simulink model "Ghost_f234"  (Simulink 8.1)
settings: Solver=ode1  StartTime=0.0  StopTime=inf  FixedStep=Ts  MaxStep=1e-3  RelTol=1e-3
PostLoadFcn:
  | NREL_Mode=1; BANSHEE_init;
InitFcn:
  | NREL_Mode=1; BANSHEE_init;
undefined symbols (not defined in the file): CBID, communications_lib, DER_REL, F0, F2, F3, F4, Feeder2_lib, Feeder3_lib, Feeder4_lib, generic_ethernet_cb, Left, relay_housing_lib, SM_UtilityService, SS_COMMUNICATION, SS_F2_RELAY_HOUSING, SS_F3_RELAY_HOUSING, SS_Feeder2, SS_Feeder3, SS_Feeder4, Stim, Ts, type, utility_service_lib, V
libraries: simulink x80, relay_modbus_lib x80, breaker_lib x46, rtio_generic_modbus x45, cables_lib x30, rtlab x22, Load_lib x21, powerlib x20, transformer_lib x19, ssn_lib x13, artemis x6, BESS_lib x4
(part 5 of 6)

== system Ghost_f234/SS_Feeder3/NGCHP_Generator ==
  note: This shall be modbus inputs
  ModbusIn : Inport
  ModbusIn1 : Inport  Port=2
  console : Inport  Port=3
  Heat Load MBtu/hrs : Inport  Port=4
  testseq : Inport  Port=5
  Bus Creator : BusCreator
  Bus Creator2 : BusCreator  Inputs=6
  Bus Creator4 : BusCreator  Inputs=3
  Bus Selector1 : BusSelector  OutputSignals=relay_out  OutputAsBus=on
  Bus Selector2 : BusSelector  OutputSignals=ModbusEnable
  Bus Selector21 : BusSelector  OutputSignals=ModbusFromSC.Ctrl,ModbusFromSC.PCmd,ModbusFromSC.QCmd,ModbusFromSC.VoltCmd,ModbusFromSC.FreqCmd,ModbusFromSC.signal6,ModbusFromSC.signal7,ModbusFromSC.signal8  OutputAsBus=on
  Bus Selector3 : BusSelector  OutputSignals=CHP_SIM_Cmds
  Bus Selector4 : BusSelector  OutputSignals=fault
  Bus Selector5 : BusSelector  OutputSignals=gen2
  Bus Selector6 : BusSelector  OutputSignals=Heat_Recovered_MBtu_hr
  Bus Selector7 : BusSelector  OutputSignals=TempActual,HeatFromBoiler MBtu/hr,CHPHeatContribution MBtu/hr,Thermal data.Heat_Recovered_MBtu_hr,Thermal data.CO2_lbm_hr,Boiler_Nm^3/hr ,Boiler lbm/hr CO2
  Bus to Vector : BusToVector
  CHPThermalModel : CHP_Model_lib/CHPThermalModel  SIM_HIL=SIM_HIL
  Demux : Demux  Outputs=2
  GCB : breaker_lib/Breaker  Ts=Ts  mech_delay=cb_mech_delay
  GenSet : NREL_Diesel_Genset_lib/GenSet  GenSel=3.5MVA natural gas generator
  Generic_Relay : relay_modbus_lib/Generic_Relay_v2_1  Ts=Ts  relay_settings=[DER_REL(CBID.GEN2,:)]
  Mux1 : Mux  Inputs=7
  SimGenCtrl : NREL_Diesel_Genset_lib/Simulated Generator Controller  GenSel=3.5MVA natural gas generator
  Switch : Switch  Criteria=u2 > Threshold  Threshold=0.5
  Gen2 A : PMIOPort  Port=1  Side=Right
  Gen2 B : PMIOPort  Port=2  Side=Right
  Gen2 C : PMIOPort  Port=3  Side=Right
  ModbusOut : Outport
  ModbusOutCHP : Outport  Port=2
  Gen_meas : Outport  Port=3
  wires:
  SimGenCtrl/9 -> Generic_Relay/2  "Logic_trip"
  SimGenCtrl/1 -> ModbusOut/1
  SimGenCtrl/8 -> GenSet/6
  SimGenCtrl/7 -> GenSet/5
  SimGenCtrl/3 -> GenSet/1
  SimGenCtrl/4 -> GenSet/2
  SimGenCtrl/5 -> GenSet/3
  SimGenCtrl/6 -> GenSet/4
  GenSet/1 -> Bus Creator/3  "gen"
  Bus Creator4/1 -> Bus Creator/4, Bus Selector1/1, SimGenCtrl/2  "cb"
  console/1 -> Bus Selector21/1, Bus Selector2/1, Bus Selector3/1
  Bus Selector2/1 -> Switch/2  "<ModbusEnable>"
  ModbusIn/1 -> Switch/1
  Bus Selector21/1 -> Bus to Vector/1
  Bus to Vector/1 -> Switch/3
  Switch/1 -> SimGenCtrl/1
  GCB/1 -> Generic_Relay/1, Bus Creator4/3  "cb_meas"
  Generic_Relay/1 -> Bus Creator4/1  "relay_out"
  Generic_Relay/2 -> Bus Creator4/2  "relay_meas"
  Bus Creator/1 -> Gen_meas/1
  SimGenCtrl/2 -> Bus Creator/2  "ctrl"
  GenSet/2 -> [HeatRec_MBtuhr]
  Bus Selector7/6 -> Mux1/6  "<Boiler_Nm^3/hr >"
  Bus Selector7/7 -> Mux1/7  "<Boiler lbm/hr CO2 >"
  CHPThermalModel/5 -> Bus Creator2/6
  CHPThermalModel/4 -> Bus Creator2/5
  Bus Selector7/3 -> Mux1/3  "<CHPHeatContribution MBtu/hr>"
  CHPThermalModel/1 -> Bus Creator2/2  "TempActual"
  Demux/2 -> CHPThermalModel/4
  CHPThermalModel/2 -> Bus Creator2/3
  Bus Selector7/2 -> Mux1/2  "<HeatFromBoiler MBtu/hr>"
  Bus Selector7/5 -> Mux1/5  "<CO2_lbm_hr>"
  Bus Selector7/4 -> Mux1/4  "<Heat_Recovered_MBtu_hr>"
  Bus Selector7/1 -> Mux1/1  "<TempActual>"
  Heat Load MBtu/hrs/1 -> CHPThermalModel/2
  Mux1/1 -> ModbusOutCHP/1
  Demux/1 -> CHPThermalModel/3
  CHPThermalModel/3 -> Bus Creator2/4
  [HeatRec_MBtuhr] -> Bus Creator2/1, Bus Selector6/1  "Thermal data"
  ModbusIn1/1 -> Demux/1
  Bus Selector6/1 -> CHPThermalModel/1  "<Heat_Recovered_MBtu_hr>"
  Bus Creator2/1 -> Bus Creator/1, Bus Selector7/1  "CHPData"
  Bus Selector3/1 -> CHPThermalModel/5  "<CHP_SIM_Cmds>"
  testseq/1 -> Bus Selector4/1
  Bus Selector4/1 -> Bus Selector5/1  "<fault>"
  Bus Selector5/1 -> SimGenCtrl/3  "<gen2>"
  Bus Selector1/1 -> GCB/1  "<relay_out>"
  connections:
  Gen2 A/RConn1 -- GCB/RConn1
  GCB/RConn2 -- Gen2 B/RConn1
  Gen2 C/RConn1 -- GCB/RConn3
  GenSet/RConn1 -- GCB/LConn1
  GenSet/RConn2 -- GCB/LConn2
  GenSet/RConn3 -- GCB/LConn3

== system Ghost_f234/SS_Feeder4/Diesel_Generator ==
  note: This shall be modbus inputs
  ModbusIn : Inport
  console : Inport  Port=2
  testseq : Inport  Port=3
  phil_meas : Inport  Port=4
  Bus Creator : BusCreator  Inputs=3
  Bus Creator4 : BusCreator  Inputs=3
  Bus Selector1 : BusSelector  OutputSignals=relay_out
  Bus Selector2 : BusSelector  OutputSignals=ModbusEnable
  Bus Selector21 : BusSelector  OutputSignals=ModbusFromSC.Ctrl,ModbusFromSC.PCmd,ModbusFromSC.QCmd,ModbusFromSC.VoltCmd,ModbusFromSC.FreqCmd,ModbusFromSC.signal6,ModbusFromSC.signal7,ModbusFromSC.signal8  OutputAsBus=on
  Bus Selector3 : BusSelector  OutputSignals=fault
  Bus Selector4 : BusSelector  OutputSignals=gen3
  Bus Selector5 : BusSelector  OutputSignals=GEN3_meas,PHIL_Enabled
  Bus to Vector : BusToVector
  GCB : breaker_lib/Breaker  Ts=Ts  mech_delay=cb_mech_delay
  GenSet : NREL_Diesel_Genset_lib/GenSet  GenSel=80kVA diesel generator
  Generic_Relay : relay_modbus_lib/Generic_Relay_v2_1  Ts=Ts  relay_settings=[DER_REL(CBID.GEN3,:)]
  SimGenCtrl : NREL_Diesel_Genset_lib/Simulated Generator Controller  GenSel=80kVA diesel generator
  Switch : Switch  Criteria=u2 > Threshold  Threshold=0.5
  Switch1 : Switch  Threshold=0.5
  Terminator : Terminator
  Gen2 A : PMIOPort  Port=1  Side=Right
  Gen2 B : PMIOPort  Port=2  Side=Right
  Gen2 C : PMIOPort  Port=3  Side=Right
  ModbusOut : Outport
  Gen3 meas : Outport  Port=2
  wires:
  GenSet/2 -> Terminator/1
  SimGenCtrl/2 -> Bus Creator/1  "ctrl"
  Bus Creator/1 -> Gen3 meas/1
  Generic_Relay/2 -> Bus Creator4/2  "relay_meas"
  Generic_Relay/1 -> Bus Creator4/1  "relay_out"
  Switch/1 -> SimGenCtrl/1
  Bus to Vector/1 -> Switch/3
  Bus Selector21/1 -> Bus to Vector/1
  ModbusIn/1 -> Switch/1
  Bus Selector2/1 -> Switch/2  "<ModbusEnable>"
  console/1 -> Bus Selector2/1, Bus Selector21/1
  Bus Creator4/1 -> SimGenCtrl/2, Bus Selector1/1, Bus Creator/3  "cb"
  GenSet/1 -> Bus Creator/2  "gen"
  SimGenCtrl/6 -> GenSet/4
  SimGenCtrl/5 -> GenSet/3
  SimGenCtrl/4 -> GenSet/2
  SimGenCtrl/3 -> GenSet/1
  SimGenCtrl/7 -> GenSet/5
  SimGenCtrl/8 -> GenSet/6
  SimGenCtrl/1 -> ModbusOut/1
  SimGenCtrl/9 -> Generic_Relay/2
  testseq/1 -> Bus Selector3/1
  Bus Selector3/1 -> Bus Selector4/1  "<fault>"
  Bus Selector4/1 -> SimGenCtrl/3  "<gen3>"
  phil_meas/1 -> Bus Selector5/1
  [CB_meas] -> Switch1/3
  Bus Selector5/1 -> Switch1/1  "<GEN3_meas>"
  Bus Selector5/2 -> Switch1/2  "<PHIL_Enabled>"
  GCB/1 -> [CB_meas]  "cb_meas"
  Switch1/1 -> Bus Creator4/3, Generic_Relay/1  "cb_meas"
  Bus Selector1/1 -> GCB/1  "<relay_out>"
  connections:
  GenSet/RConn3 -- GCB/LConn3
  GenSet/RConn2 -- GCB/LConn2
  GenSet/RConn1 -- GCB/LConn1
  Gen2 C/RConn1 -- GCB/RConn3
  GCB/RConn2 -- Gen2 B/RConn1
  Gen2 A/RConn1 -- GCB/RConn1

== system Ghost_f234/SS_Feeder4/ESS2 ==
  modbus_in : Inport
  console : Inport  Port=2
  testseq : Inport  Port=3
  phil_meas : Inport  Port=4
  Bus Creator4 : BusCreator  Inputs=3
  Bus Selector : BusSelector  OutputSignals=cb_ctrl
  Bus Selector1 : BusSelector  OutputSignals=ModbusEnable
  Bus Selector2 : BusSelector  OutputSignals=fault
  Bus Selector20 : BusSelector  OutputSignals=relay_ctrl
  Bus Selector21 : BusSelector  OutputSignals=ModbusFromSC.Ctrl,ModbusFromSC.PCmd,ModbusFromSC.QCmd,ModbusFromSC.VoltCmd,ModbusFromSC.FreqCmd,ModbusFromSC.signal6,ModbusFromSC.signal7,ModbusFromSC.signal8  OutputAsBus=on
  Bus Selector3 : BusSelector  OutputSignals=ess2
  Bus Selector4 : BusSelector  OutputSignals=Tuning
  Bus Selector5 : BusSelector  OutputSignals=ESS2_meas,PHIL_Enabled
  Bus to Vector : BusToVector
  Constant : Constant  Value=0
  ESS2 : BESS_lib/NREL_BESS  InvType=ESS Inverter  Sn=250  Vn=480  b_Vdc_nom=1000  b_kWh=60  b_esr=0.1  r_I_max=3  Tc=Ts  MbusPrecInc=on  ExtTuningEna=on
  F4_CB_3 : breaker_lib/Breaker  Ts=Ts  mech_delay=cb_mech_delay
  Generic_Relay : relay_modbus_lib/Generic_Relay_v2_1  Ts=Ts  relay_settings=[DER_REL(CBID.ESS2,:)]
  Switch : Switch  Criteria=u2 > Threshold  Threshold=0.5
  Switch1 : Switch  Threshold=0.5
  A : PMIOPort  Port=1  Side=Right
  B : PMIOPort  Port=2  Side=Right
  C : PMIOPort  Port=3  Side=Right
  modbus_out : Outport
  meas : Outport  Port=2
  wires:
  Bus Creator4/1 -> ESS2/5
  Generic_Relay/2 -> Bus Creator4/2  "relay_meas"
  ESS2/2 -> meas/1  "PV_meas"
  Generic_Relay/1 -> Bus Creator4/1  "relay_out"
  Bus Selector20/1 -> Generic_Relay/2  "<relay_ctrl>"
  console/1 -> Bus Selector4/1, Bus Selector1/1, Bus Selector21/1
  Bus Selector1/1 -> Switch/2  "<ModbusEnable>"
  ESS2/1 -> modbus_out/1
  modbus_in/1 -> Switch/1
  Bus Selector21/1 -> Bus to Vector/1
  Switch/1 -> ESS2/1
  ESS2/3 -> Bus Selector20/1, Bus Selector/1
  Bus to Vector/1 -> Switch/3
  Constant/1 -> ESS2/3
  testseq/1 -> Bus Selector2/1
  Bus Selector2/1 -> Bus Selector3/1  "<fault>"
  Bus Selector3/1 -> ESS2/4  "<ess2>"
  phil_meas/1 -> Bus Selector5/1
  [CB_meas] -> Switch1/3
  Bus Selector5/1 -> Switch1/1  "<ESS2_meas>"
  Bus Selector5/2 -> Switch1/2  "<PHIL_Enabled>"
  Switch1/1 -> Generic_Relay/1, Bus Creator4/3  "cb_meas"
  F4_CB_3/1 -> [CB_meas]  "cb_meas"
  Bus Selector/1 -> F4_CB_3/1  "<cb_ctrl>"
  Bus Selector4/1 -> ESS2/2  "<Tuning>"
  connections:
  F4_CB_3/RConn2 -- B/RConn1
  ESS2/RConn2 -- F4_CB_3/LConn2
  ESS2/RConn3 -- F4_CB_3/LConn3
  ESS2/RConn1 -- F4_CB_3/LConn1
  A/RConn1 -- F4_CB_3/RConn1
  F4_CB_3/RConn3 -- C/RConn1

== system Ghost_f234/SS_Feeder4/PV2 ==
  modbus_in : Inport
  console : Inport  Port=2
  testseq : Inport  Port=3
  phil_meas : Inport  Port=4
  Bus Creator : BusCreator  Inputs=5
  Bus Creator1 : BusCreator  Inputs=7
  Bus Creator4 : BusCreator  Inputs=3
  Bus Selector : BusSelector  OutputSignals=cb_ctrl
  Bus Selector1 : BusSelector  OutputSignals=ModbusEnable
  Bus Selector2 : BusSelector  OutputSignals=pv.insolation2
  Bus Selector20 : BusSelector  OutputSignals=relay_ctrl
  Bus Selector21 : BusSelector  OutputSignals=ModbusFromSC.Ctrl,ModbusFromSC.PCmd,ModbusFromSC.QCmd,ModbusFromSC.VoltCmd,ModbusFromSC.FreqCmd,ModbusFromSC.signal6,ModbusFromSC.signal7,ModbusFromSC.signal8  OutputAsBus=on
  Bus Selector3 : BusSelector  OutputSignals=fault
  Bus Selector4 : BusSelector  OutputSignals=pv2
  Bus Selector5 : BusSelector  OutputSignals=PV2_meas,PHIL_Enabled,Magna_meas
  Bus Selector6 : BusSelector  OutputSignals=Tuning
  Bus Selector7 : BusSelector  OutputSignals=Vdc
  Bus Selector8 : BusSelector  OutputSignals=Inverter,CB_meas,Battery,status_word,Logic_trip,raw
  Bus Selector9 : BusSelector  OutputSignals=Vdc,Idc,Pdc
  Bus to Vector : BusToVector
  Constant1 : Constant  Value=25
  Constant2 : Constant  Value=31
  Constant3 : Constant  Value=36
  Constant4 : Constant
  Constant5 : Constant  Value=0
  Constant6 : Constant  Value=590
  F4_CB_4 : breaker_lib/Breaker  Ts=Ts  mech_delay=cb_mech_delay
  Gain : Gain  Gain=1000
  Generic_Relay : relay_modbus_lib/Generic_Relay_v2_1  Ts=Ts  relay_settings=[DER_REL(CBID.PV2,:)]
  Inverter : BESS_lib/NREL_BESS  InvType=PV Inverter  Sn=100  Vn=480  b_Vdc_nom=1000  b_kWh=1  b_esr=0.1  r_I_max=1.2  Tc=Ts  MbusPrecInc=on  ExtTuningEna=on
  PV model : Subsystem
  Switch : Switch  Criteria=u2 > Threshold  Threshold=0.5
  Switch1 : Switch  Threshold=0.5
  Terminator : Terminator
  A : PMIOPort  Port=1  Side=Right
  B : PMIOPort  Port=2  Side=Right
  C : PMIOPort  Port=3  Side=Right
  modbus_out : Outport
  meas : Outport  Port=2
  wires:
  Inverter/3 -> Bus Selector20/1, Bus Selector/1
  Switch/1 -> Inverter/1
  Bus to Vector/1 -> Switch/3
  modbus_in/1 -> Switch/1
  Inverter/1 -> modbus_out/1
  Bus Selector20/1 -> Generic_Relay/2  "<relay_ctrl>"
  Generic_Relay/1 -> Bus Creator4/1  "relay_out"
  Inverter/2 -> Bus Selector8/1  "PV_meas"
  Generic_Relay/2 -> Bus Creator4/2  "relay_meas"
  Bus Creator4/1 -> Inverter/5
  testseq/1 -> Bus Selector3/1, Bus Selector2/1
  console/1 -> Bus Selector6/1, Bus Selector21/1, Bus Selector1/1
  Bus Selector1/1 -> Switch/2  "<ModbusEnable>"
  Bus Selector21/1 -> Bus to Vector/1
  Bus Selector2/1 -> Gain/1, Inverter/3  "<insolation2>"
  Bus Selector3/1 -> Bus Selector4/1  "<fault>"
  Bus Selector4/1 -> Inverter/4  "<pv2>"
  phil_meas/1 -> Bus Selector5/1
  [CB_meas] -> Switch1/3
  Bus Selector5/1 -> Switch1/1  "<PV2_meas>"
  Bus Selector5/2 -> Switch1/2  "<PHIL_Enabled>"
  Switch1/1 -> Bus Creator4/3, Generic_Relay/1  "cb_meas"
  F4_CB_4/1 -> [CB_meas]  "cb_meas"
  Bus Selector/1 -> F4_CB_4/1  "<cb_ctrl>"
  Bus Selector6/1 -> Inverter/2  "<Tuning>"
  Constant1/1 -> PV model/3(Tamb)
  Constant3/1 -> PV model/6(ParallelN)
  Constant2/1 -> PV model/5(SeriesN)
  Constant4/1 -> PV model/7(Imin)
  Constant5/1 -> PV model/2(Idc_meas)
  Gain/1 -> PV model/4(POA_Insolation)
  Bus Selector5/3 -> Bus Selector9/1, Bus Selector7/1  "<Magna_meas>"
  Bus Selector7/1 -> PV model/1(Vdc_meas)  "<Vdc>"
  PV model/1(Vpv_set) -> Terminator/1
  PV model/2(Ipv_set) -> Bus Creator/5  "Iref"
  Constant6/1 -> Bus Creator/4  "Vref"
  Bus Creator/1 -> Bus Creator1/7  "pv_phil"
  Bus Selector8/6 -> Bus Creator1/6  "<raw>"
  Bus Selector8/5 -> Bus Creator1/5  "<Logic_trip>"
  Bus Selector8/4 -> Bus Creator1/4  "<status_word>"
  Bus Selector8/3 -> Bus Creator1/3  "<Battery>"
  Bus Selector8/2 -> Bus Creator1/2  "<CB_meas>"
  Bus Selector8/1 -> Bus Creator1/1  "<Inverter>"
  Bus Creator1/1 -> meas/1
  Bus Selector9/2 -> Bus Creator/2  "<Idc>"
  Bus Selector9/3 -> Bus Creator/3  "<Pdc>"
  Bus Selector9/1 -> Bus Creator/1  "<Vdc>"
  connections:
  F4_CB_4/RConn3 -- C/RConn1
  A/RConn1 -- F4_CB_4/RConn1
  Inverter/RConn1 -- F4_CB_4/LConn1
  Inverter/RConn3 -- F4_CB_4/LConn3
  Inverter/RConn2 -- F4_CB_4/LConn2
  F4_CB_4/RConn2 -- B/RConn1

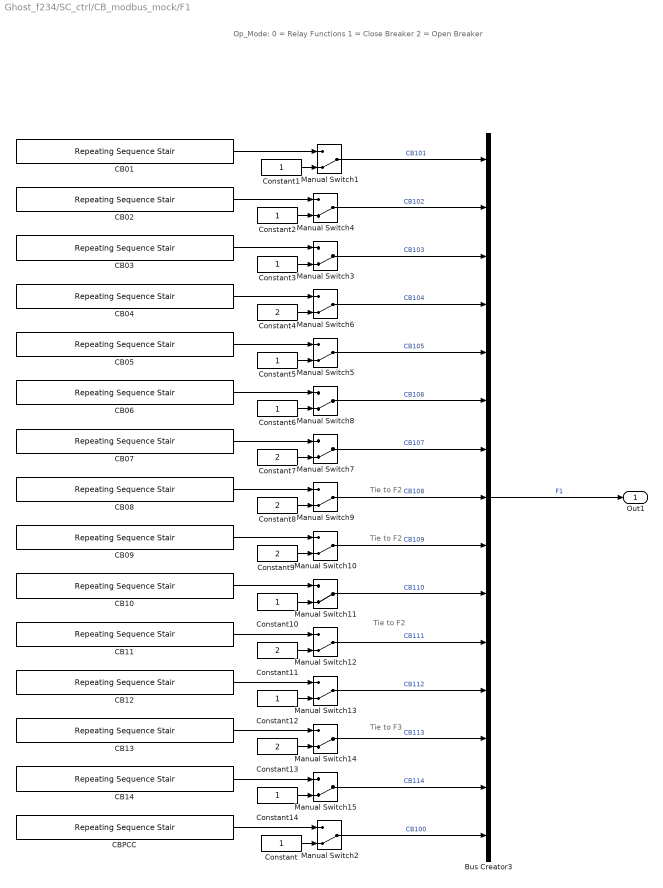
== system Ghost_f234/SC_ctrl/CB_modbus_mock/F1 ==
  note: Tie to F2
  note: Tie to F2
  note: Op_Mode:
      | 0 = Relay Functions
      | 1 = Close Breaker
      | 2 = Open Breaker
  note: Tie to F2
  note: Tie to F3
  Bus Creator3 : BusCreator  Inputs=15
  CB01 : simulink/Sources/Repeating Sequence Stair  OutValues=Stim.CB.CB101  tsamp=[Stim.Ts Ts]  OutMin=[]  OutMax=[]  OutDataTypeStr=Inherit: Inherit via back propagation  OutDataType=fixdt(0,8)  ConRadixGroup=Best Precision: Vector-wise  OutScaling=2^-12
  CB02 : simulink/Sources/Repeating Sequence Stair  OutValues=Stim.CB.CB102  tsamp=[Stim.Ts Ts]  OutMin=[]  OutMax=[]  OutDataTypeStr=Inherit: Inherit via back propagation  OutDataType=fixdt(0,8)  ConRadixGroup=Best Precision: Vector-wise  OutScaling=2^-12
  CB03 : simulink/Sources/Repeating Sequence Stair  OutValues=Stim.CB.CB103  tsamp=[Stim.Ts Ts]  OutMin=[]  OutMax=[]  OutDataTypeStr=Inherit: Inherit via back propagation  OutDataType=fixdt(0,8)  ConRadixGroup=Best Precision: Vector-wise  OutScaling=2^-12
  CB04 : simulink/Sources/Repeating Sequence Stair  OutValues=Stim.CB.CB104  tsamp=[Stim.Ts Ts]  OutMin=[]  OutMax=[]  OutDataTypeStr=Inherit: Inherit via back propagation  OutDataType=fixdt(0,8)  ConRadixGroup=Best Precision: Vector-wise  OutScaling=2^-12
  CB05 : simulink/Sources/Repeating Sequence Stair  OutValues=Stim.CB.CB105  tsamp=[Stim.Ts Ts]  OutMin=[]  OutMax=[]  OutDataTypeStr=Inherit: Inherit via back propagation  OutDataType=fixdt(0,8)  ConRadixGroup=Best Precision: Vector-wise  OutScaling=2^-12
  CB06 : simulink/Sources/Repeating Sequence Stair  OutValues=Stim.CB.CB106  tsamp=[Stim.Ts Ts]  OutMin=[]  OutMax=[]  OutDataTypeStr=Inherit: Inherit via back propagation  OutDataType=fixdt(0,8)  ConRadixGroup=Best Precision: Vector-wise  OutScaling=2^-12
  CB07 : simulink/Sources/Repeating Sequence Stair  OutValues=Stim.CB.CB107  tsamp=[Stim.Ts Ts]  OutMin=[]  OutMax=[]  OutDataTypeStr=Inherit: Inherit via back propagation  OutDataType=fixdt(0,8)  ConRadixGroup=Best Precision: Vector-wise  OutScaling=2^-12
  CB08 : simulink/Sources/Repeating Sequence Stair  OutValues=Stim.CB.CB108  tsamp=[Stim.Ts Ts]  OutMin=[]  OutMax=[]  OutDataTypeStr=Inherit: Inherit via back propagation  OutDataType=fixdt(0,8)  ConRadixGroup=Best Precision: Vector-wise  OutScaling=2^-12
  CB09 : simulink/Sources/Repeating Sequence Stair  OutValues=Stim.CB.CB109  tsamp=[Stim.Ts Ts]  OutMin=[]  OutMax=[]  OutDataTypeStr=Inherit: Inherit via back propagation  OutDataType=fixdt(0,8)  ConRadixGroup=Best Precision: Vector-wise  OutScaling=2^-12
  CB10 : simulink/Sources/Repeating Sequence Stair  OutValues=Stim.CB.CB110  tsamp=[Stim.Ts Ts]  OutMin=[]  OutMax=[]  OutDataTypeStr=Inherit: Inherit via back propagation  OutDataType=fixdt(0,8)  ConRadixGroup=Best Precision: Vector-wise  OutScaling=2^-12
  CB11 : simulink/Sources/Repeating Sequence Stair  OutValues=Stim.CB.CB111  tsamp=[Stim.Ts Ts]  OutMin=[]  OutMax=[]  OutDataTypeStr=Inherit: Inherit via back propagation  OutDataType=fixdt(0,8)  ConRadixGroup=Best Precision: Vector-wise  OutScaling=2^-12
  CB12 : simulink/Sources/Repeating Sequence Stair  OutValues=Stim.CB.CB112  tsamp=[Stim.Ts Ts]  OutMin=[]  OutMax=[]  OutDataTypeStr=Inherit: Inherit via back propagation  OutDataType=fixdt(0,8)  ConRadixGroup=Best Precision: Vector-wise  OutScaling=2^-12
  CB13 : simulink/Sources/Repeating Sequence Stair  OutValues=Stim.CB.CB113  tsamp=[Stim.Ts Ts]  OutMin=[]  OutMax=[]  OutDataTypeStr=Inherit: Inherit via back propagation  OutDataType=fixdt(0,8)  ConRadixGroup=Best Precision: Vector-wise  OutScaling=2^-12
  CB14 : simulink/Sources/Repeating Sequence Stair  OutValues=Stim.CB.CB114  tsamp=[Stim.Ts Ts]  OutMin=[]  OutMax=[]  OutDataTypeStr=Inherit: Inherit via back propagation  OutDataType=fixdt(0,8)  ConRadixGroup=Best Precision: Vector-wise  OutScaling=2^-12
  CBPCC : simulink/Sources/Repeating Sequence Stair  OutValues=Stim.CB.CB100  tsamp=[Stim.Ts Ts]  OutMin=[]  OutMax=[]  OutDataTypeStr=Inherit: Inherit via back propagation  OutDataType=fixdt(0,8)  ConRadixGroup=Best Precision: Vector-wise  OutScaling=2^-12
  Constant{,1..3,5..6,10,12,14} (9 alike) : Constant
  Constant{4,7..9,11,13} (6 alike) : Constant  Value=2
  Manual Switch{1..15} (15 alike) : ManualSwitch  CurrentSetting=0
  Out1 : Outport
  wires:
  CB08/1 -> Manual Switch9/1
  Constant8/1 -> Manual Switch9/2
  Constant9/1 -> Manual Switch10/2
  Manual Switch9/1 -> Bus Creator3/8  "CB108"
  CB02/1 -> Manual Switch4/1
  Constant1/1 -> Manual Switch1/2
  Constant7/1 -> Manual Switch7/2
  Constant6/1 -> Manual Switch8/2
  CB07/1 -> Manual Switch7/1
  CB09/1 -> Manual Switch10/1
  Constant2/1 -> Manual Switch4/2
  CB06/1 -> Manual Switch8/1
  CB05/1 -> Manual Switch5/1
  Constant4/1 -> Manual Switch6/2
  Constant5/1 -> Manual Switch5/2
  CB04/1 -> Manual Switch6/1
  Manual Switch10/1 -> Bus Creator3/9  "CB109"
  Manual Switch8/1 -> Bus Creator3/6  "CB106"
  Manual Switch5/1 -> Bus Creator3/5  "CB105"
  Manual Switch6/1 -> Bus Creator3/4  "CB104"
  Manual Switch4/1 -> Bus Creator3/2  "CB102"
  Manual Switch1/1 -> Bus Creator3/1  "CB101"
  Manual Switch3/1 -> Bus Creator3/3  "CB103"
  Manual Switch7/1 -> Bus Creator3/7  "CB107"
  Manual Switch2/1 -> Bus Creator3/15  "CB100"
  Constant/1 -> Manual Switch2/2
  CBPCC/1 -> Manual Switch2/1
  CB01/1 -> Manual Switch1/1
  Bus Creator3/1 -> Out1/1  "F1"
  CB03/1 -> Manual Switch3/1
  Constant3/1 -> Manual Switch3/2
  Constant10/1 -> Manual Switch11/2
  CB10/1 -> Manual Switch11/1
  Manual Switch11/1 -> Bus Creator3/10  "CB110"
  Constant11/1 -> Manual Switch12/2
  CB11/1 -> Manual Switch12/1
  Manual Switch12/1 -> Bus Creator3/11  "CB111"
  Constant12/1 -> Manual Switch13/2
  CB12/1 -> Manual Switch13/1
  Manual Switch13/1 -> Bus Creator3/12  "CB112"
  Constant13/1 -> Manual Switch14/2
  CB13/1 -> Manual Switch14/1
  Manual Switch14/1 -> Bus Creator3/13  "CB113"
  Constant14/1 -> Manual Switch15/2
  CB14/1 -> Manual Switch15/1
  Manual Switch15/1 -> Bus Creator3/14  "CB114"

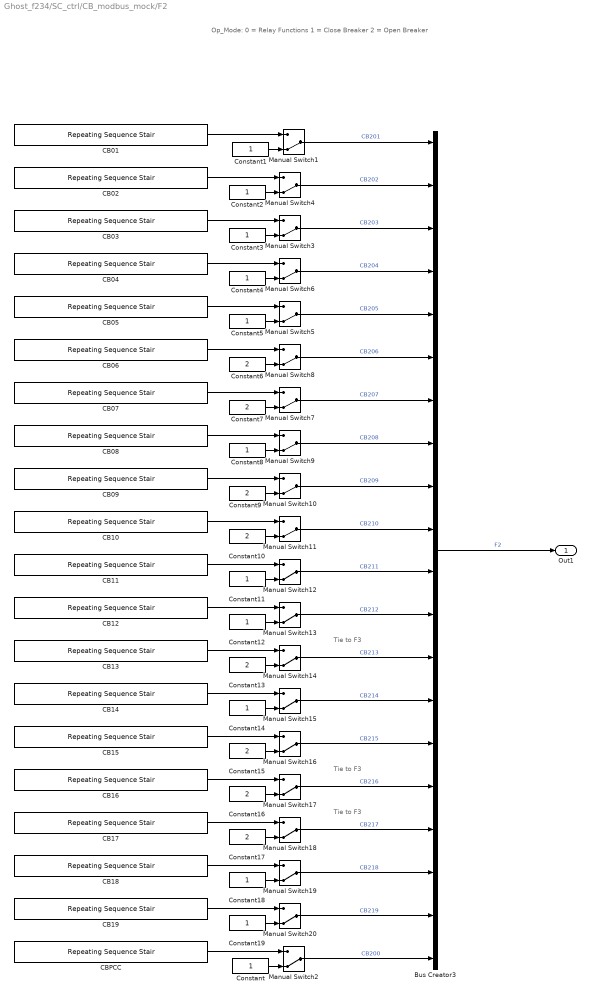
== system Ghost_f234/SC_ctrl/CB_modbus_mock/F2 ==
  note: Tie to F3
  note: Op_Mode:
      | 0 = Relay Functions
      | 1 = Close Breaker
      | 2 = Open Breaker
  note: Tie to F3
  note: Tie to F3
  Bus Creator3 : BusCreator  Inputs=20
  CB01 : simulink/Sources/Repeating Sequence Stair  OutValues=Stim.CB.CB201  tsamp=[Stim.Ts Ts]  OutMin=[]  OutMax=[]  OutDataTypeStr=Inherit: Inherit via back propagation  OutDataType=fixdt(0,8)  ConRadixGroup=Best Precision: Vector-wise  OutScaling=2^-12
  CB02 : simulink/Sources/Repeating Sequence Stair  OutValues=Stim.CB.CB202  tsamp=[Stim.Ts Ts]  OutMin=[]  OutMax=[]  OutDataTypeStr=Inherit: Inherit via back propagation  OutDataType=fixdt(0,8)  ConRadixGroup=Best Precision: Vector-wise  OutScaling=2^-12
  CB03 : simulink/Sources/Repeating Sequence Stair  OutValues=Stim.CB.CB203  tsamp=[Stim.Ts Ts]  OutMin=[]  OutMax=[]  OutDataTypeStr=Inherit: Inherit via back propagation  OutDataType=fixdt(0,8)  ConRadixGroup=Best Precision: Vector-wise  OutScaling=2^-12
  CB04 : simulink/Sources/Repeating Sequence Stair  OutValues=Stim.CB.CB204  tsamp=[Stim.Ts Ts]  OutMin=[]  OutMax=[]  OutDataTypeStr=Inherit: Inherit via back propagation  OutDataType=fixdt(0,8)  ConRadixGroup=Best Precision: Vector-wise  OutScaling=2^-12
  CB05 : simulink/Sources/Repeating Sequence Stair  OutValues=Stim.CB.CB205  tsamp=[Stim.Ts Ts]  OutMin=[]  OutMax=[]  OutDataTypeStr=Inherit: Inherit via back propagation  OutDataType=fixdt(0,8)  ConRadixGroup=Best Precision: Vector-wise  OutScaling=2^-12
  CB06 : simulink/Sources/Repeating Sequence Stair  OutValues=Stim.CB.CB206  tsamp=[Stim.Ts Ts]  OutMin=[]  OutMax=[]  OutDataTypeStr=Inherit: Inherit via back propagation  OutDataType=fixdt(0,8)  ConRadixGroup=Best Precision: Vector-wise  OutScaling=2^-12
  CB07 : simulink/Sources/Repeating Sequence Stair  OutValues=Stim.CB.CB207  tsamp=[Stim.Ts Ts]  OutMin=[]  OutMax=[]  OutDataTypeStr=Inherit: Inherit via back propagation  OutDataType=fixdt(0,8)  ConRadixGroup=Best Precision: Vector-wise  OutScaling=2^-12
  CB08 : simulink/Sources/Repeating Sequence Stair  OutValues=Stim.CB.CB208  tsamp=[Stim.Ts Ts]  OutMin=[]  OutMax=[]  OutDataTypeStr=Inherit: Inherit via back propagation  OutDataType=fixdt(0,8)  ConRadixGroup=Best Precision: Vector-wise  OutScaling=2^-12
  CB09 : simulink/Sources/Repeating Sequence Stair  OutValues=Stim.CB.CB209  tsamp=[Stim.Ts Ts]  OutMin=[]  OutMax=[]  OutDataTypeStr=Inherit: Inherit via back propagation  OutDataType=fixdt(0,8)  ConRadixGroup=Best Precision: Vector-wise  OutScaling=2^-12
  CB10 : simulink/Sources/Repeating Sequence Stair  OutValues=Stim.CB.CB210  tsamp=[Stim.Ts Ts]  OutMin=[]  OutMax=[]  OutDataTypeStr=Inherit: Inherit via back propagation  OutDataType=fixdt(0,8)  ConRadixGroup=Best Precision: Vector-wise  OutScaling=2^-12
  CB11 : simulink/Sources/Repeating Sequence Stair  OutValues=Stim.CB.CB211  tsamp=[Stim.Ts Ts]  OutMin=[]  OutMax=[]  OutDataTypeStr=Inherit: Inherit via back propagation  OutDataType=fixdt(0,8)  ConRadixGroup=Best Precision: Vector-wise  OutScaling=2^-12
  CB12 : simulink/Sources/Repeating Sequence Stair  OutValues=Stim.CB.CB212  tsamp=[Stim.Ts Ts]  OutMin=[]  OutMax=[]  OutDataTypeStr=Inherit: Inherit via back propagation  OutDataType=fixdt(0,8)  ConRadixGroup=Best Precision: Vector-wise  OutScaling=2^-12
  CB13 : simulink/Sources/Repeating Sequence Stair  OutValues=Stim.CB.CB213  tsamp=[Stim.Ts Ts]  OutMin=[]  OutMax=[]  OutDataTypeStr=Inherit: Inherit via back propagation  OutDataType=fixdt(0,8)  ConRadixGroup=Best Precision: Vector-wise  OutScaling=2^-12
  CB14 : simulink/Sources/Repeating Sequence Stair  OutValues=Stim.CB.CB214  tsamp=[Stim.Ts Ts]  OutMin=[]  OutMax=[]  OutDataTypeStr=Inherit: Inherit via back propagation  OutDataType=fixdt(0,8)  ConRadixGroup=Best Precision: Vector-wise  OutScaling=2^-12
  CB15 : simulink/Sources/Repeating Sequence Stair  OutValues=Stim.CB.CB215  tsamp=[Stim.Ts Ts]  OutMin=[]  OutMax=[]  OutDataTypeStr=Inherit: Inherit via back propagation  OutDataType=fixdt(0,8)  ConRadixGroup=Best Precision: Vector-wise  OutScaling=2^-12
  CB16 : simulink/Sources/Repeating Sequence Stair  OutValues=Stim.CB.CB216  tsamp=[Stim.Ts Ts]  OutMin=[]  OutMax=[]  OutDataTypeStr=Inherit: Inherit via back propagation  OutDataType=fixdt(0,8)  ConRadixGroup=Best Precision: Vector-wise  OutScaling=2^-12
  CB17 : simulink/Sources/Repeating Sequence Stair  OutValues=Stim.CB.CB217  tsamp=[Stim.Ts Ts]  OutMin=[]  OutMax=[]  OutDataTypeStr=Inherit: Inherit via back propagation  OutDataType=fixdt(0,8)  ConRadixGroup=Best Precision: Vector-wise  OutScaling=2^-12
  CB18 : simulink/Sources/Repeating Sequence Stair  OutValues=Stim.CB.CB218  tsamp=[Stim.Ts Ts]  OutMin=[]  OutMax=[]  OutDataTypeStr=Inherit: Inherit via back propagation  OutDataType=fixdt(0,8)  ConRadixGroup=Best Precision: Vector-wise  OutScaling=2^-12
  CB19 : simulink/Sources/Repeating Sequence Stair  OutValues=Stim.CB.CB219  tsamp=[Stim.Ts Ts]  OutMin=[]  OutMax=[]  OutDataTypeStr=Inherit: Inherit via back propagation  OutDataType=fixdt(0,8)  ConRadixGroup=Best Precision: Vector-wise  OutScaling=2^-12
  CBPCC : simulink/Sources/Repeating Sequence Stair  OutValues=Stim.CB.CB200  tsamp=[Stim.Ts Ts]  OutMin=[]  OutMax=[]  OutDataTypeStr=Inherit: Inherit via back propagation  OutDataType=fixdt(0,8)  ConRadixGroup=Best Precision: Vector-wise  OutScaling=2^-12
  Constant{,1..5,8,11..12,14,18..19} (12 alike) : Constant
  Constant{6..7,9..10,13,15..17} (8 alike) : Constant  Value=2
  Manual Switch{1..20} (20 alike) : ManualSwitch  CurrentSetting=0
  Out1 : Outport
  wires:
  Manual Switch15/1 -> Bus Creator3/14  "CB214"
  CB14/1 -> Manual Switch15/1
  Constant14/1 -> Manual Switch15/2
  Manual Switch14/1 -> Bus Creator3/13  "CB213"
  CB13/1 -> Manual Switch14/1
  Constant13/1 -> Manual Switch14/2
  Manual Switch13/1 -> Bus Creator3/12  "CB212"
  CB12/1 -> Manual Switch13/1
  Constant12/1 -> Manual Switch13/2
  Manual Switch12/1 -> Bus Creator3/11  "CB211"
  CB11/1 -> Manual Switch12/1
  Constant11/1 -> Manual Switch12/2
  Manual Switch11/1 -> Bus Creator3/10  "CB210"
  CB10/1 -> Manual Switch11/1
  Constant10/1 -> Manual Switch11/2
  Constant3/1 -> Manual Switch3/2
  CB03/1 -> Manual Switch3/1
  Bus Creator3/1 -> Out1/1  "F2"
  CB01/1 -> Manual Switch1/1
  CBPCC/1 -> Manual Switch2/1
  Constant/1 -> Manual Switch2/2
  Manual Switch2/1 -> Bus Creator3/20  "CB200"
  Manual Switch7/1 -> Bus Creator3/7  "CB207"
  Manual Switch3/1 -> Bus Creator3/3  "CB203"
  Manual Switch1/1 -> Bus Creator3/1  "CB201"
  Manual Switch4/1 -> Bus Creator3/2  "CB202"
  Manual Switch6/1 -> Bus Creator3/4  "CB204"
  Manual Switch5/1 -> Bus Creator3/5  "CB205"
  Manual Switch8/1 -> Bus Creator3/6  "CB206"
  Manual Switch10/1 -> Bus Creator3/9  "CB209"
  CB04/1 -> Manual Switch6/1
  Constant5/1 -> Manual Switch5/2
  Constant4/1 -> Manual Switch6/2
  CB05/1 -> Manual Switch5/1
  CB06/1 -> Manual Switch8/1
  Constant2/1 -> Manual Switch4/2
  CB09/1 -> Manual Switch10/1
  CB07/1 -> Manual Switch7/1
  Constant6/1 -> Manual Switch8/2
  Constant7/1 -> Manual Switch7/2
  Constant1/1 -> Manual Switch1/2
  CB02/1 -> Manual Switch4/1
  Manual Switch9/1 -> Bus Creator3/8  "CB208"
  Constant9/1 -> Manual Switch10/2
  Constant8/1 -> Manual Switch9/2
  CB08/1 -> Manual Switch9/1
  Manual Switch20/1 -> Bus Creator3/19  "CB219"
  CB19/1 -> Manual Switch20/1
  Constant19/1 -> Manual Switch20/2
  Manual Switch19/1 -> Bus Creator3/18  "CB218"
  CB18/1 -> Manual Switch19/1
  Constant18/1 -> Manual Switch19/2
  Manual Switch18/1 -> Bus Creator3/17  "CB217"
  CB17/1 -> Manual Switch18/1
  Constant17/1 -> Manual Switch18/2
  Manual Switch17/1 -> Bus Creator3/16  "CB216"
  CB16/1 -> Manual Switch17/1
  Constant16/1 -> Manual Switch17/2
  Manual Switch16/1 -> Bus Creator3/15  "CB215"
  CB15/1 -> Manual Switch16/1
  Constant15/1 -> Manual Switch16/2

== system Ghost_f234/SC_ctrl/CB_modbus_mock/F3 ==
  note: Tie to F4 (PHIL)
  note: Op_Mode:
      | 0 = Relay Functions
      | 1 = Close Breaker
      | 2 = Open Breaker
  Bus Creator3 : BusCreator  Inputs=11
  CB01 : simulink/Sources/Repeating Sequence Stair  OutValues=Stim.CB.CB301  tsamp=[Stim.Ts Ts]  OutMin=[]  OutMax=[]  OutDataTypeStr=Inherit: Inherit via back propagation  OutDataType=fixdt(0,8)  ConRadixGroup=Best Precision: Vector-wise  OutScaling=2^-12
  CB02 : simulink/Sources/Repeating Sequence Stair  OutValues=Stim.CB.CB302  tsamp=[Stim.Ts Ts]  OutMin=[]  OutMax=[]  OutDataTypeStr=Inherit: Inherit via back propagation  OutDataType=fixdt(0,8)  ConRadixGroup=Best Precision: Vector-wise  OutScaling=2^-12
  CB03 : simulink/Sources/Repeating Sequence Stair  OutValues=Stim.CB.CB303  tsamp=[Stim.Ts Ts]  OutMin=[]  OutMax=[]  OutDataTypeStr=Inherit: Inherit via back propagation  OutDataType=fixdt(0,8)  ConRadixGroup=Best Precision: Vector-wise  OutScaling=2^-12
  CB04 : simulink/Sources/Repeating Sequence Stair  OutValues=Stim.CB.CB304  tsamp=[Stim.Ts Ts]  OutMin=[]  OutMax=[]  OutDataTypeStr=Inherit: Inherit via back propagation  OutDataType=fixdt(0,8)  ConRadixGroup=Best Precision: Vector-wise  OutScaling=2^-12
  CB05 : simulink/Sources/Repeating Sequence Stair  OutValues=Stim.CB.CB305  tsamp=[Stim.Ts Ts]  OutMin=[]  OutMax=[]  OutDataTypeStr=Inherit: Inherit via back propagation  OutDataType=fixdt(0,8)  ConRadixGroup=Best Precision: Vector-wise  OutScaling=2^-12
  CB06 : simulink/Sources/Repeating Sequence Stair  OutValues=Stim.CB.CB306  tsamp=[Stim.Ts Ts]  OutMin=[]  OutMax=[]  OutDataTypeStr=Inherit: Inherit via back propagation  OutDataType=fixdt(0,8)  ConRadixGroup=Best Precision: Vector-wise  OutScaling=2^-12
  CB07 : simulink/Sources/Repeating Sequence Stair  OutValues=Stim.CB.CB307  tsamp=[Stim.Ts Ts]  OutMin=[]  OutMax=[]  OutDataTypeStr=Inherit: Inherit via back propagation  OutDataType=fixdt(0,8)  ConRadixGroup=Best Precision: Vector-wise  OutScaling=2^-12
  CB08 : simulink/Sources/Repeating Sequence Stair  OutValues=Stim.CB.CB308  tsamp=[Stim.Ts Ts]  OutMin=[]  OutMax=[]  OutDataTypeStr=Inherit: Inherit via back propagation  OutDataType=fixdt(0,8)  ConRadixGroup=Best Precision: Vector-wise  OutScaling=2^-12
  CB09 : simulink/Sources/Repeating Sequence Stair  OutValues=Stim.CB.CB309  tsamp=[Stim.Ts Ts]  OutMin=[]  OutMax=[]  OutDataTypeStr=Inherit: Inherit via back propagation  OutDataType=fixdt(0,8)  ConRadixGroup=Best Precision: Vector-wise  OutScaling=2^-12
  CB10 : simulink/Sources/Repeating Sequence Stair  OutValues=Stim.CB.CB310  tsamp=[Stim.Ts Ts]  OutMin=[]  OutMax=[]  OutDataTypeStr=Inherit: Inherit via back propagation  OutDataType=fixdt(0,8)  ConRadixGroup=Best Precision: Vector-wise  OutScaling=2^-12
  CBPCC : simulink/Sources/Repeating Sequence Stair  OutValues=Stim.CB.CB300  tsamp=[Stim.Ts Ts]  OutMin=[]  OutMax=[]  OutDataTypeStr=Inherit: Inherit via back propagation  OutDataType=fixdt(0,8)  ConRadixGroup=Best Precision: Vector-wise  OutScaling=2^-12
  Constant{,1..7,9} (9 alike) : Constant
  Constant10 : Constant  Value=2
  Constant8 : Constant  Value=2
  Manual Switch{1..11} (11 alike) : ManualSwitch  CurrentSetting=0
  Out1 : Outport
  wires:
  CB08/1 -> Manual Switch9/1
  Constant8/1 -> Manual Switch9/2
  Constant9/1 -> Manual Switch10/2
  Manual Switch9/1 -> Bus Creator3/8  "CB308"
  CB02/1 -> Manual Switch4/1
  Constant1/1 -> Manual Switch1/2
  Constant7/1 -> Manual Switch7/2
  Constant6/1 -> Manual Switch8/2
  CB07/1 -> Manual Switch7/1
  CB09/1 -> Manual Switch10/1
  Constant2/1 -> Manual Switch4/2
  CB06/1 -> Manual Switch8/1
  CB05/1 -> Manual Switch5/1
  Constant4/1 -> Manual Switch6/2
  Constant5/1 -> Manual Switch5/2
  CB04/1 -> Manual Switch6/1
  Manual Switch10/1 -> Bus Creator3/9  "CB309"
  Manual Switch8/1 -> Bus Creator3/6  "CB306"
  Manual Switch5/1 -> Bus Creator3/5  "CB305"
  Manual Switch6/1 -> Bus Creator3/4  "CB304"
  Manual Switch4/1 -> Bus Creator3/2  "CB302"
  Manual Switch1/1 -> Bus Creator3/1  "CB301"
  Manual Switch3/1 -> Bus Creator3/3  "CB303"
  Manual Switch7/1 -> Bus Creator3/7  "CB307"
  Manual Switch2/1 -> Bus Creator3/11  "CB300"
  Constant/1 -> Manual Switch2/2
  CBPCC/1 -> Manual Switch2/1
  CB01/1 -> Manual Switch1/1
  Bus Creator3/1 -> Out1/1  "F3"
  CB03/1 -> Manual Switch3/1
  Constant3/1 -> Manual Switch3/2
  Constant10/1 -> Manual Switch11/2
  CB10/1 -> Manual Switch11/1
  Manual Switch11/1 -> Bus Creator3/10  "CB310"

== system Ghost_f234/SC_ctrl/CB_modbus_mock/F4 ==
  note: Copyright © 2017 the Alliance for Sustainable Energy, LLC
      |
      | The above copyright notice and this permission notice shall be included in all copies or substantial portions of the Software.
      |
      | THE SOFTWARE IS PROVIDED "AS IS", WITHOUT WARRANTY OF ANY KIND, EXPRESS OR IMPLIED, INCLUDING
      | BUT NOT LIMITED TO THE WARRANTIES OF MERCHANTABILITY, FITNESS FOR A PARTICULAR PURPOSE AND
      | NONINFRINGEMENT. IN NO EVENT SHALL THE AUTHORS OR COPYRIGHT HOLDERS BE LIABLE FOR ANY CLAIM,
      |  DAMAGES OR OTHER LIABILITY, WHETHER IN AN ACTION OF CONTRACT, TORT OR OTHERWISE, ARISING FROM,
      | OUT OF OR IN CONNECTION WITH THE SOFTWARE OR THE USE OR OTHER DEALINGS IN THE SOFTWARE
  note: Op_Mode:
      | 0 = Relay Functions
      | 1 = Close Breaker
      | 2 = Open Breaker
  Bus Creator3 : BusCreator  Inputs=6
  CB401 : simulink/Sources/Repeating Sequence Stair  OutValues=Stim.CB.CB401  tsamp=[Stim.Ts Ts]  OutMin=[]  OutMax=[]  OutDataTypeStr=Inherit: Inherit via back propagation  OutDataType=fixdt(0,8)  ConRadixGroup=Best Precision: Vector-wise  OutScaling=2^-12
  CB402 : simulink/Sources/Repeating Sequence Stair  OutValues=Stim.CB.CB402  tsamp=[Stim.Ts Ts]  OutMin=[]  OutMax=[]  OutDataTypeStr=Inherit: Inherit via back propagation  OutDataType=fixdt(0,8)  ConRadixGroup=Best Precision: Vector-wise  OutScaling=2^-12
  CB403 : simulink/Sources/Repeating Sequence Stair  OutValues=Stim.CB.CB403  tsamp=[Stim.Ts Ts]  OutMin=[]  OutMax=[]  OutDataTypeStr=Inherit: Inherit via back propagation  OutDataType=fixdt(0,8)  ConRadixGroup=Best Precision: Vector-wise  OutScaling=2^-12
  CB404 : simulink/Sources/Repeating Sequence Stair  OutValues=Stim.CB.CB404  tsamp=[Stim.Ts Ts]  OutMin=[]  OutMax=[]  OutDataTypeStr=Inherit: Inherit via back propagation  OutDataType=fixdt(0,8)  ConRadixGroup=Best Precision: Vector-wise  OutScaling=2^-12
  CB405 : simulink/Sources/Repeating Sequence Stair  OutValues=Stim.CB.CB405  tsamp=[Stim.Ts Ts]  OutMin=[]  OutMax=[]  OutDataTypeStr=Inherit: Inherit via back propagation  OutDataType=fixdt(0,8)  ConRadixGroup=Best Precision: Vector-wise  OutScaling=2^-12
  CB406 : simulink/Sources/Repeating Sequence Stair  OutValues=Stim.CB.CB406  tsamp=[Stim.Ts Ts]  OutMin=[]  OutMax=[]  OutDataTypeStr=Inherit: Inherit via back propagation  OutDataType=fixdt(0,8)  ConRadixGroup=Best Precision: Vector-wise  OutScaling=2^-12
  Constant : Constant  Value=2
  Constant{1..5} (5 alike) : Constant  Value=0
  Manual Switch{1,3..6} (5 alike) : ManualSwitch
  Manual Switch2 : ManualSwitch  CurrentSetting=0
  Out1 : Outport
  wires:
  Constant5/1 -> Manual Switch6/2
  CB406/1 -> Manual Switch6/1
  Constant4/1 -> Manual Switch5/2
  CB405/1 -> Manual Switch5/1
  Constant3/1 -> Manual Switch4/2
  CB404/1 -> Manual Switch4/1
  Constant2/1 -> Manual Switch3/2
  CB403/1 -> Manual Switch3/1
  Constant1/1 -> Manual Switch1/2
  Manual Switch4/1 -> Bus Creator3/4  "CB404"
  Manual Switch3/1 -> Bus Creator3/3  "CB403"
  Manual Switch5/1 -> Bus Creator3/5  "CB405"
  Manual Switch1/1 -> Bus Creator3/2  "CB402"
  CB402/1 -> Manual Switch1/1
  Manual Switch6/1 -> Bus Creator3/6  "CB406"
  Manual Switch2/1 -> Bus Creator3/1  "CB401"
  Constant/1 -> Manual Switch2/2
  CB401/1 -> Manual Switch2/1
  Bus Creator3/1 -> Out1/1  "F4"

== system Ghost_f234/SC_ctrl/PV1 control/Tuning ==
  Bus Creator : BusCreator  Inputs=5
  Constant : Constant  Value=2  SampleTime=[Stim.Ts Ts]
  Constant1 : Constant  Value=0.6e-3  SampleTime=[Stim.Ts Ts]
  Constant2 : Constant  Value=180  SampleTime=[Stim.Ts Ts]
  Constant3 : Constant  Value=3200  SampleTime=[Stim.Ts Ts]
  Constant4 : Constant  SampleTime=[Stim.Ts Ts]
  Tuning : Outport
  wires:
  Constant4/1 -> Bus Creator/5  "vff_ena"
  Constant3/1 -> Bus Creator/4  "pll_ki"
  Constant2/1 -> Bus Creator/3  "pll_kp"
  Constant1/1 -> Bus Creator/2  "csi_Ti"
  Constant/1 -> Bus Creator/1  "csi_kp"
  Bus Creator/1 -> Tuning/1

== system Ghost_f234/SC_ctrl/PV2 control/Tuning ==
  Bus Creator : BusCreator  Inputs=5
  Constant : Constant  Value=2  SampleTime=[Stim.Ts Ts]
  Constant1 : Constant  Value=0.6e-3  SampleTime=[Stim.Ts Ts]
  Constant2 : Constant  Value=180  SampleTime=[Stim.Ts Ts]
  Constant3 : Constant  Value=3200  SampleTime=[Stim.Ts Ts]
  Constant4 : Constant  SampleTime=[Stim.Ts Ts]
  Tuning : Outport
  wires:
  Constant4/1 -> Bus Creator/5  "vff_ena"
  Constant3/1 -> Bus Creator/4  "pll_ki"
  Constant2/1 -> Bus Creator/3  "pll_kp"
  Constant1/1 -> Bus Creator/2  "csi_Ti"
  Constant/1 -> Bus Creator/1  "csi_kp"
  Bus Creator/1 -> Tuning/1

== system Ghost_f234/SC_ctrl/SOC1 control/Tuning ==
  Bus Creator : BusCreator  Inputs=5
  Constant : Constant  Value=2  SampleTime=[Stim.Ts Ts]
  Constant1 : Constant  Value=0.6e-3  SampleTime=[Stim.Ts Ts]
  Constant2 : Constant  Value=180  SampleTime=[Stim.Ts Ts]
  Constant3 : Constant  Value=3200  SampleTime=[Stim.Ts Ts]
  Constant4 : Constant  SampleTime=[Stim.Ts Ts]
  Tuning : Outport
  wires:
  Constant4/1 -> Bus Creator/5  "vff_ena"
  Constant3/1 -> Bus Creator/4  "pll_ki"
  Constant2/1 -> Bus Creator/3  "pll_kp"
  Constant1/1 -> Bus Creator/2  "csi_Ti"
  Constant/1 -> Bus Creator/1  "csi_kp"
  Bus Creator/1 -> Tuning/1

== system Ghost_f234/SC_ctrl/SOC2 control/Tuning ==
  Bus Creator : BusCreator  Inputs=5
  Constant : Constant  Value=2  SampleTime=[Stim.Ts Ts]
  Constant1 : Constant  Value=0.6e-3  SampleTime=[Stim.Ts Ts]
  Constant2 : Constant  Value=180  SampleTime=[Stim.Ts Ts]
  Constant3 : Constant  Value=3200  SampleTime=[Stim.Ts Ts]
  Constant4 : Constant  SampleTime=[Stim.Ts Ts]
  Tuning : Outport
  wires:
  Constant4/1 -> Bus Creator/5  "vff_ena"
  Constant3/1 -> Bus Creator/4  "pll_ki"
  Constant2/1 -> Bus Creator/3  "pll_kp"
  Constant1/1 -> Bus Creator/2  "csi_Ti"
  Constant/1 -> Bus Creator/1  "csi_kp"
  Bus Creator/1 -> Tuning/1

== system Ghost_f234/SC_ctrl/TestSequenceGen/Time_ms ==
  Constant4 : Constant  Value=10
  Sum : Sum  Inputs=++|
  Unit Delay : UnitDelay  SampleTime=10e-3
  Simtime_ms : Outport
  wires:
  Sum/1 -> Simtime_ms/1, Unit Delay/1
  Constant4/1 -> Sum/2
  Unit Delay/1 -> Sum/1

== system Ghost_f234/SC_ctrl/TestSequenceGen/uint32_2_uint16 ==
  In1 : Inport
  Data Type Conversion : DataTypeConversion  OutDataTypeStr=uint32
  Data Type Conversion1 : DataTypeConversion  OutDataTypeStr=double
  Data Type Conversion2 : DataTypeConversion  OutDataTypeStr=double
  Extract Bits : simulink/Logic and Bit Operations/Extract Bits  bitsToExtract=Upper half  numBits=8  bitIdxRange=[0 7]  outScalingMode=Treat bit field as an integer
  Extract Bits1 : simulink/Logic and Bit Operations/Extract Bits  bitsToExtract=Lower half  numBits=8  bitIdxRange=[0 7]  outScalingMode=Preserve fixed-point scaling
  Mux : Mux  Inputs=2
  Out1 : Outport
  wires:
  Mux/1 -> Out1/1
  Extract Bits/1 -> Data Type Conversion1/1
  In1/1 -> Data Type Conversion/1
  Data Type Conversion/1 -> Extract Bits1/1, Extract Bits/1
  Data Type Conversion2/1 -> Mux/1
  Data Type Conversion1/1 -> Mux/2
  Extract Bits1/1 -> Data Type Conversion2/1

== system Ghost_f234/SS_COMMUNICATION/MGC_controller/Subsystem ==
  Bus Selector18 : BusSelector  OutputSignals=F3_CB_CTRL
  Bus Selector19 : BusSelector  OutputSignals=signal11
  Bus Selector20 : BusSelector  OutputSignals=F2_CB_CTRL
  Bus Selector21 : BusSelector  OutputSignals=signal20
  Constant : Constant  Value=0
  Mux : Mux  Inputs=3
  Out1 : Outport
  wires:
  Bus Selector20/1 -> Bus Selector21/1  "<F2_CB_CTRL>"
  Bus Selector19/1 -> Mux/3  "<signal11>"
  Bus Selector18/1 -> Bus Selector19/1  "<F3_CB_CTRL>"
  Mux/1 -> Out1/1
  Bus Selector21/1 -> Mux/2  "<signal20>"
  [F3_RELAY_OUT] -> Bus Selector18/1
  [F2_RELAY_OUT] -> Bus Selector20/1
  Constant/1 -> Mux/1

== system Ghost_f234/SS_COMMUNICATION/Misc_data/Subsystem ==
  In1 : Inport
  Bus Selector28 : BusSelector  OutputSignals=F2.LOAD_DATA.F2_I3.kw,F2.LOAD_DATA.F2_I4.kw,F2.LOAD_DATA.F2_I5.kw,F3.LOAD_DATA.F3_I6.kw,F4.LOAD_DATA.F4_I7.kw,F4.LOAD_DATA.F4_I8.kw,F2.LOAD_DATA.F2_P2.kw,F2.LOAD_DATA.F2_P3.kw,F3.LOAD_DATA.F3_P4.kw,F2.LOAD_DATA.F2_P5.kw,F3.LOAD_DATA.F3_P6.kw,F4.LOAD_DATA.F4_P7.kw,F4.LOAD_DATA.F4_P8.kw,F2.LOAD_DATA.F2_C3.kw,F2.LOAD_DATA.F2_C4.kw,F3.LOAD_DATA.F3_C5.kw,F3.LOAD_DATA.F3_C6.kw,F4.LOAD_DATA.F4_C7.kw,F4.LOAD_DATA.F4_C8.kw,F4.LOAD_DATA.F4_C9.kw
  Constant : Constant  Value=0
  Mux : Mux  Inputs=25
  Out1 : Outport
  wires:
  In1/1 -> Bus Selector28/1
  Bus Selector28/14 -> Mux/19  "<kw>"
  Bus Selector28/1 -> Mux/3  "<kw>"
  Bus Selector28/9 -> Mux/12  "<kw>"
  Bus Selector28/16 -> Mux/21  "<kw>"
  Bus Selector28/7 -> Mux/10  "<kw>"
  Bus Selector28/15 -> Mux/20  "<kw>"
  Bus Selector28/8 -> Mux/11  "<kw>"
  Bus Selector28/5 -> Mux/7  "<kw>"
  Bus Selector28/10 -> Mux/13  "<kw>"
  Bus Selector28/17 -> Mux/22  "<kw>"
  Bus Selector28/19 -> Mux/24  "<kw>"
  Bus Selector28/18 -> Mux/23  "<kw>"
  Bus Selector28/20 -> Mux/25  "<kw>"
  Bus Selector28/2 -> Mux/4  "<kw>"
  Bus Selector28/13 -> Mux/16  "<kw>"
  Bus Selector28/4 -> Mux/6  "<kw>"
  Bus Selector28/6 -> Mux/8  "<kw>"
  Bus Selector28/12 -> Mux/15  "<kw>"
  Bus Selector28/3 -> Mux/5  "<kw>"
  Bus Selector28/11 -> Mux/14  "<kw>"
  Mux/1 -> Out1/1
  Constant/1 -> Mux/17, Mux/18, Mux/9, Mux/2, Mux/1

== system Ghost_f234/SS_COMMUNICATION/Misc_data/Subsystem1 ==
  In1 : Inport
  Bus Selector29 : BusSelector  OutputSignals=F2.LOAD_DATA.F2_I3.VRMSLL,F2.LOAD_DATA.F2_I4.VRMSLL,F2.LOAD_DATA.F2_I5.VRMSLL,F3.LOAD_DATA.F3_I6.VRMSLL,F4.LOAD_DATA.F4_I7.VRMSLL,F4.LOAD_DATA.F4_I8.VRMSLL,F2.LOAD_DATA.F2_P2.VRMSLL,F2.LOAD_DATA.F2_P3.VRMSLL,F3.LOAD_DATA.F3_P4.VRMSLL,F2.LOAD_DATA.F2_P5.VRMSLL,F3.LOAD_DATA.F3_P6.VRMSLL,F4.LOAD_DATA.F4_P7.VRMSLL,F4.LOAD_DATA.F4_P8.VRMSLL,F2.LOAD_DATA.F2_C3.VRMSLL,F2.LOAD_DATA.F2_C4.VRMSLL,F3.LOAD_DATA.F3_C5.VRMSLL,F3.LOAD_DATA.F3_C6.VRMSLL,F4.LOAD_DATA.F4_C7.VRMSLL,F4.LOAD_DATA.F4_C8.VRMSLL,F4.LOAD_DATA.F4_C9.VRMSLL
  Constant : Constant  Value=0
  Mux : Mux  Inputs=25
  Out1 : Outport
  wires:
  Mux/1 -> Out1/1
  In1/1 -> Bus Selector29/1
  Bus Selector29/8 -> Mux/11  "<VRMSLL>"
  Bus Selector29/9 -> Mux/12  "<VRMSLL>"
  Bus Selector29/7 -> Mux/10  "<VRMSLL>"
  Bus Selector29/5 -> Mux/7  "<VRMSLL>"
  Bus Selector29/6 -> Mux/8  "<VRMSLL>"
  Bus Selector29/3 -> Mux/5  "<VRMSLL>"
  Bus Selector29/4 -> Mux/6  "<VRMSLL>"
  Bus Selector29/2 -> Mux/4  "<VRMSLL>"
  Bus Selector29/1 -> Mux/3  "<VRMSLL>"
  Bus Selector29/20 -> Mux/25  "<VRMSLL>"
  Bus Selector29/19 -> Mux/24  "<VRMSLL>"
  Bus Selector29/18 -> Mux/23  "<VRMSLL>"
  Bus Selector29/17 -> Mux/22  "<VRMSLL>"
  Bus Selector29/16 -> Mux/21  "<VRMSLL>"
  Bus Selector29/15 -> Mux/20  "<VRMSLL>"
  Bus Selector29/14 -> Mux/19  "<VRMSLL>"
  Bus Selector29/13 -> Mux/16  "<VRMSLL>"
  Bus Selector29/12 -> Mux/15  "<VRMSLL>"
  Bus Selector29/11 -> Mux/14  "<VRMSLL>"
  Bus Selector29/10 -> Mux/13  "<VRMSLL>"
  Constant/1 -> Mux/1, Mux/2, Mux/9, Mux/18, Mux/17

== system Ghost_f234/SS_COMMUNICATION/NREL UDP Data - Formatted Packets/Number of seconds of recording ==
  Compare To Constant1 : simulink/Logic and Bit Operations/Compare To Constant  relop=>=  const=time_s  OutDataTypeStr=boolean
  Increment : Subsystem
  Integrator : Integrator  ExternalReset=rising
  Memory : Memory
  Slope : Constant
  file suffix : Outport
  wires:
  Slope/1 -> Integrator/1
  Integrator/1 -> Compare To Constant1/1
  Compare To Constant1/1 -> Memory/1, Increment/Trigger  "limit reached"
  Memory/1 -> Integrator/2
  Increment/1(Out1) -> file suffix/1

== system Ghost_f234/SS_COMMUNICATION/NREL UDP Data - Formatted Packets/Trigg_machine ==
  Write : Inport
  Odd : Inport  Port=2
  Even : Inport  Port=3
  Bitwise Operator : simulink/Logic and Bit Operations/Bitwise Operator  logicop=AND  UseBitMask=off  NumInputPorts=2  BitMask=bin2dec('11011001')  BitMaskRealWorld=Stored Integer
  Bitwise Operator1 : simulink/Logic and Bit Operations/Bitwise Operator  logicop=AND  UseBitMask=off  NumInputPorts=2  BitMask=bin2dec('11011001')  BitMaskRealWorld=Stored Integer
  Data Type Conversion : DataTypeConversion
  Data Type Conversion1 : DataTypeConversion
  Double2uint8 : DataTypeConversion
  Trig_odd : Outport
  Trig_even : Outport  Port=2
  wires:
  Double2uint8/1 -> Bitwise Operator1/1, Bitwise Operator/2
  Write/1 -> Double2uint8/1
  Odd/1 -> Bitwise Operator/1
  Data Type Conversion1/1 -> Trig_even/1
  Data Type Conversion/1 -> Trig_odd/1
  Even/1 -> Bitwise Operator1/2
  Bitwise Operator1/1 -> Data Type Conversion1/1
  Bitwise Operator/1 -> Data Type Conversion/1

== system Ghost_f234/SS_COMMUNICATION/NREL UDP Data - Formatted Packets/isOddOrEven ==
  note: Si cette différence est égale à 0, c'est que le
      | nombre en entrée est pair, sinon c'est qu'il est impair.
  note: Effectuer la différence entre le nombre en entrée,
      | et sa moitié arrondie multipliée par 2.
  Index : Inport
  Compare To Zero : simulink/Logic and Bit Operations/Compare To Zero  relop=~=  OutDataTypeStr=boolean  ZeroCross=off
  Compare To Zero1 : simulink/Logic and Bit Operations/Compare To Zero  relop===  OutDataTypeStr=boolean  ZeroCross=off
  Constant3 : Constant  Value=2
  Divide : Product  Inputs=*/  OutDataTypeStr=double
  Produit : Product  Inputs=**  OutDataTypeStr=double
  Rounding Function : Rounding
  Sum : Sum  Inputs=|+-
  isOdd : Outport
  isEven : Outport  Port=2
  wires:
  Compare To Zero1/1 -> isEven/1
  Compare To Zero/1 -> isOdd/1
  Sum/1 -> Compare To Zero1/1, Compare To Zero/1
  Produit/1 -> Sum/2
  Rounding Function/1 -> Produit/1
  Index/1 -> Sum/1, Divide/1
  Divide/1 -> Rounding Function/1
  Constant3/1 -> Produit/2, Divide/2

== system Ghost_f234/SS_COMMUNICATION/NREL UDP Data - Formatted Packets/uint32_2_uint16 ==
  In1 : Inport
  Data Type Conversion : DataTypeConversion  OutDataTypeStr=uint32
  Data Type Conversion1 : DataTypeConversion  OutDataTypeStr=double
  Data Type Conversion2 : DataTypeConversion  OutDataTypeStr=double
  Extract Bits : simulink/Logic and Bit Operations/Extract Bits  bitsToExtract=Upper half  numBits=8  bitIdxRange=[0 7]  outScalingMode=Treat bit field as an integer
  Extract Bits1 : simulink/Logic and Bit Operations/Extract Bits  bitsToExtract=Lower half  numBits=8  bitIdxRange=[0 7]  outScalingMode=Preserve fixed-point scaling
  Mux : Mux  Inputs=2
  Out1 : Outport
  wires:
  Extract Bits1/1 -> Data Type Conversion2/1
  Data Type Conversion1/1 -> Mux/2
  Data Type Conversion2/1 -> Mux/1
  Data Type Conversion/1 -> Extract Bits/1, Extract Bits1/1
  In1/1 -> Data Type Conversion/1
  Extract Bits/1 -> Data Type Conversion1/1
  Mux/1 -> Out1/1

== system Ghost_f234/SS_COMMUNICATION/Relay_data/ExtractF2 ==
  In1 : Inport
  Bus Selector{1..5,48..53,56,58..64} (19 alike) : BusSelector  OutputSignals=m.kw,m.kvar,m.Vpu,m.Hz,m.status  OutputAsBus=on
  Bus Selector47 : BusSelector  OutputSignals=F2_CB_1,F2_CB_2,F2_CB_3,F2_CB_4,F2_CB_5,F2_CB_6,F2_CB_7,F2_CB_8,F2_CB_9,F2_CB_10,F2_CB_11,F2_CB_12,F2_CB_13,F2_CB_14,F2_CB_15,F2_CB_16,F2_CB_17,F2_CB_18,F2_CB_19
  Mux13 : Mux  Inputs=19
  Out1 : Outport
  wires:
  Bus Selector63/1 -> Mux13/13
  Bus Selector61/1 -> Mux13/3
  Bus Selector62/1 -> Mux13/12
  Bus Selector59/1 -> Mux13/10
  Bus Selector47/5 -> Bus Selector51/1  "<F2_CB_5>"
  Bus Selector47/10 -> Bus Selector59/1  "<F2_CB_10>"
  Bus Selector49/1 -> Mux13/2
  Bus Selector47/14 -> Bus Selector64/1  "<F2_CB_14>"
  Bus Selector47/2 -> Bus Selector49/1  "<F2_CB_2>"
  Bus Selector47/3 -> Bus Selector61/1  "<F2_CB_3>"
  Bus Selector47/9 -> Bus Selector58/1  "<F2_CB_9>"
  Bus Selector47/8 -> Bus Selector56/1  "<F2_CB_8>"
  Bus Selector47/12 -> Bus Selector62/1  "<F2_CB_12>"
  Bus Selector47/7 -> Bus Selector53/1  "<F2_CB_7>"
  Bus Selector64/1 -> Mux13/14
  Bus Selector47/6 -> Bus Selector52/1  "<F2_CB_6>"
  Bus Selector58/1 -> Mux13/9
  Bus Selector56/1 -> Mux13/8
  Bus Selector52/1 -> Mux13/6
  Bus Selector47/11 -> Bus Selector60/1  "<F2_CB_11>"
  Bus Selector60/1 -> Mux13/11
  Mux13/1 -> Out1/1
  In1/1 -> Bus Selector47/1
  Bus Selector50/1 -> Mux13/4
  Bus Selector47/1 -> Bus Selector48/1  "<F2_CB_1>"
  Bus Selector47/4 -> Bus Selector50/1  "<F2_CB_4>"
  Bus Selector53/1 -> Mux13/7
  Bus Selector48/1 -> Mux13/1
  Bus Selector51/1 -> Mux13/5
  Bus Selector47/13 -> Bus Selector63/1  "<F2_CB_13>"
  Bus Selector4/1 -> Mux13/18
  Bus Selector3/1 -> Mux13/17
  Bus Selector1/1 -> Mux13/15
  Bus Selector47/15 -> Bus Selector1/1  "<F2_CB_15>"
  Bus Selector47/19 -> Bus Selector5/1  "<F2_CB_19>"
  Bus Selector47/17 -> Bus Selector3/1  "<F2_CB_17>"
  Bus Selector5/1 -> Mux13/19
  Bus Selector47/16 -> Bus Selector2/1  "<F2_CB_16>"
  Bus Selector2/1 -> Mux13/16
  Bus Selector47/18 -> Bus Selector4/1  "<F2_CB_18>"
